simulink subsystem "FOC"  (R2023b)
settings: Solver=VariableStepAuto  StartTime=0.0  StopTime=10.0  RelTol=1e-3
undefined symbols (not defined in the file): NPoles, tSimMoCo
libraries: slpidlib x2
settings Model: Creator=Elio  LastModifiedBy=Elio

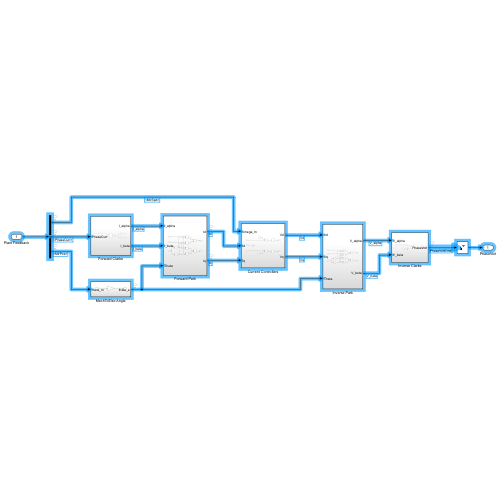
[thumbnail: Simulink's stored preview of the top-level diagram]
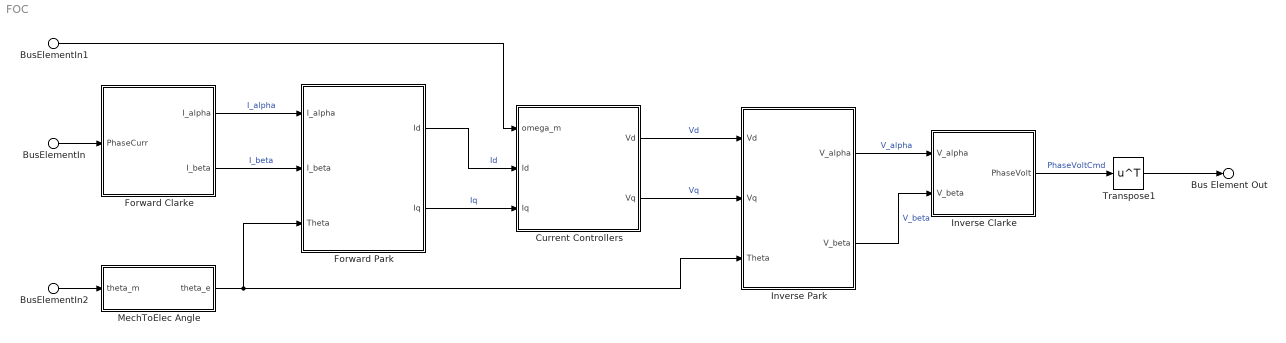
== system FOC ==
  BusElementIn1 : Inport  PortName=FOCInputs  Element=wRotorSpd
  BusElementIn : Inport  PortName=FOCInputs  Element=IPhase
  BusElementIn2 : Inport  PortName=FOCInputs  Element=aRotorMechPos
  Current Controllers : Subsystem
  Forward Clarke : Subsystem
  Forward Park : Subsystem
  Inverse Clarke : Subsystem
  Inverse Park : Subsystem
  MechToElec Angle : Subsystem
  Transpose1 : Math  Operator=transpose
  Bus Element Out : Outport  PortName=FOCCmds  Element=VPhase
  wires:
  Current Controllers/1(Vd) -> Inverse Park/1(Vd)  "Vd"
  Forward Clarke/2(I_beta) -> Forward Park/2(I_beta)  "I_beta"
  Current Controllers/2(Vq) -> Inverse Park/2(Vq)  "Vq"
  Forward Park/1(Id) -> Current Controllers/2(Id)  "Id"
  MechToElec Angle/1(theta_e) -> Forward Park/3(Theta), Inverse Park/3(Theta)
  BusElementIn/1 -> Forward Clarke/1(PhaseCurr)
  Forward Clarke/1(I_alpha) -> Forward Park/1(I_alpha)  "I_alpha"
  Inverse Park/2(V_beta) -> Inverse Clarke/2(V_beta)  "V_beta"
  Inverse Park/1(V_alpha) -> Inverse Clarke/1(V_alpha)  "V_alpha"
  Transpose1/1 -> Bus Element Out/1
  Forward Park/2(Iq) -> Current Controllers/3(Iq)  "Iq"
  Inverse Clarke/1(PhaseVolt) -> Transpose1/1  "PhaseVoltCmd"
  BusElementIn2/1 -> MechToElec Angle/1(theta_m)
  BusElementIn1/1 -> Current Controllers/1(omega_m)

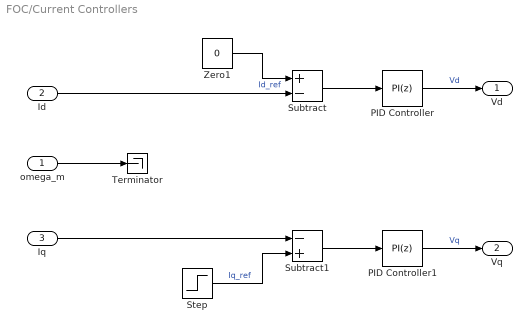
== system FOC/Current Controllers ==
  omega_m : Inport
  Id : Inport  Port=2
  Iq : Inport  Port=3
  PID Controller : slpidlib/PID Controller  Controller=PI  Form=Parallel  TimeDomain=Discrete-time  UseExternalTs=off  SampleTime=1e-5  IntegratorMethod=Forward Euler  FilterMethod=Forward Euler  ControllerParametersSource=internal  P=13.4666695236978  I=8567.48164264561  UseKiTs=off  D=0  N=100  UseFilter=on  TunerSelectOption=Transfer Function Based (PID Tuner App)  InitialConditionSource=internal  InitialConditionForIntegrator=0  InitialConditionForFilter=0  DifferentiatorICPrevScaledInput=0  ExternalReset=none  TrackingMode=off  Kt=1  LimitOutput=off  SatLimitsSource=internal  UpperSaturationLimit=inf  LowerSaturationLimit=-inf  LinearizeAsGain=on  AntiWindupMode=none  Kb=1  LimitIntegrator=off  UpperIntegratorSaturationLimit=inf  LowerIntegratorSaturationLimit=-inf  POutMin=[]  POutMax=[]  IOutMin=[]  IOutMax=[]  DOutMin=[]  DOutMax=[]  NOutMin=[]  NOutMax=[]  SumOutMin=[]  SumOutMax=[]  SaturationOutMin=[]  SaturationOutMax=[]  PParamMin=[]  PParamMax=[]  IParamMin=[]  IParamMax=[]  DParamMin=[]  DParamMax=[]  NParamMin=[]  NParamMax=[]  KbParamMin=[]  KbParamMax=[]  KtParamMin=[]  KtParamMax=[]  KbOutMin=[]  KbOutMax=[]  KtOutMin=[]  KtOutMax=[]  IntegratorOutMin=[]  IntegratorOutMax=[]  FilterOutMin=[]  FilterOutMax=[]  SumI1OutMin=[]  SumI1OutMax=[]  SumI2OutMin=[]  SumI2OutMax=[]  SumI3OutMin=[]  SumI3OutMax=[]  SumI4OutMin=[]  SumI4OutMax=[]  SumDOutMin=[]  SumDOutMax=[]  DifferentiatorOutMin=[]  DifferentiatorOutMax=[]  FilterDiffOutCoefMin=[]  FilterDiffOutCoefMax=[]  ReciprocalOutMin=[]  ReciprocalOutMax=[]  SumDenOutMin=[]  SumDenOutMax=[]  SumNumOutMin=[]  SumNumOutMax=[]  DivideOutMin=[]  DivideOutMax=[]  UdiffTsProdOutMin=[]  UdiffTsProdOutMax=[]  NTsProdOutMin=[]  NTsProdOutMax=[]  UintegralTsProdOutMin=[]  UintegralTsProdOutMax=[]  UngainTsProdOutMin=[]  UngainTsProdOutMax=[]  ClampingZeroOutDataTypeStr=Inherit: Inherit via back propagation  ClampingZeroOutMin=[]  ClampingZeroOutMax=[]  FilterDenConstantOutDataTypeStr=Inherit: Inherit via back propagation  FilterDenConstantOutMin=[]  FilterDenConstantOutMax=[]  PCopyOutDataTypeStr=Inherit: Inherit via back propagation  PCopyOutMin=[]  PCopyOutMax=[]  NCopyOutDataTypeStr=Inherit: Inherit via back propagation  NCopyOutMin=[]  NCopyOutMax=[]  IntegratorContinuousStateAttributes=''  IntegratorStateMustResolveToSignalObject=off  IntegratorRTWStateStorageClass=Auto  FilterContinuousStateAttributes=''  FilterStateMustResolveToSignalObject=off  FilterRTWStateStorageClass=Auto  ParallelPVariant=InternalParameters  IdealPVariant=Disabled  IVariant=InternalParameters  DVariant=Disabled  IntegratorVariant=Discrete  SatVariant=Disabled  AWVariant=Passthrough  PCopyVariant=Disabled  TRVariant=Disabled  FdbkBlocksVariant=Forward  IdealPFdbkVariant=Disabled  SatFdbkVariant=Disabled  DerivativeFilterVariant=Disabled  NVariant=Disabled  NCopyVariant=Disabled_SignalSpec  FilterICVariant=Disabled  IntegratorICVariant=InternalICs  ExternalResetVariant=Disabled  TRSumVariant=Passthrough  SumFdbkVariant=Disabled  SumVariant=Sum_PI  TsampFilterVariant=InternalTs  TsampNgainVariant=Passthrough  TsampIntegralVariant=Disabled_SignalSpec  ExternalSaturationOutDataTypeStr=Inherit: Same as second input
  PID Controller1 : slpidlib/PID Controller  Controller=PI  Form=Parallel  TimeDomain=Discrete-time  UseExternalTs=off  SampleTime=1e-5  IntegratorMethod=Forward Euler  FilterMethod=Forward Euler  ControllerParametersSource=internal  P=25  I=12500  UseKiTs=off  D=0  N=100  UseFilter=on  TunerSelectOption=Transfer Function Based (PID Tuner App)  InitialConditionSource=internal  InitialConditionForIntegrator=0  InitialConditionForFilter=0  DifferentiatorICPrevScaledInput=0  ExternalReset=none  TrackingMode=off  Kt=1  LimitOutput=off  SatLimitsSource=internal  UpperSaturationLimit=inf  LowerSaturationLimit=-inf  LinearizeAsGain=on  AntiWindupMode=none  Kb=1  LimitIntegrator=off  UpperIntegratorSaturationLimit=inf  LowerIntegratorSaturationLimit=-inf  POutMin=[]  POutMax=[]  IOutMin=[]  IOutMax=[]  DOutMin=[]  DOutMax=[]  NOutMin=[]  NOutMax=[]  SumOutMin=[]  SumOutMax=[]  SaturationOutMin=[]  SaturationOutMax=[]  PParamMin=[]  PParamMax=[]  IParamMin=[]  IParamMax=[]  DParamMin=[]  DParamMax=[]  NParamMin=[]  NParamMax=[]  KbParamMin=[]  KbParamMax=[]  KtParamMin=[]  KtParamMax=[]  KbOutMin=[]  KbOutMax=[]  KtOutMin=[]  KtOutMax=[]  IntegratorOutMin=[]  IntegratorOutMax=[]  FilterOutMin=[]  FilterOutMax=[]  SumI1OutMin=[]  SumI1OutMax=[]  SumI2OutMin=[]  SumI2OutMax=[]  SumI3OutMin=[]  SumI3OutMax=[]  SumI4OutMin=[]  SumI4OutMax=[]  SumDOutMin=[]  SumDOutMax=[]  DifferentiatorOutMin=[]  DifferentiatorOutMax=[]  FilterDiffOutCoefMin=[]  FilterDiffOutCoefMax=[]  ReciprocalOutMin=[]  ReciprocalOutMax=[]  SumDenOutMin=[]  SumDenOutMax=[]  SumNumOutMin=[]  SumNumOutMax=[]  DivideOutMin=[]  DivideOutMax=[]  UdiffTsProdOutMin=[]  UdiffTsProdOutMax=[]  NTsProdOutMin=[]  NTsProdOutMax=[]  UintegralTsProdOutMin=[]  UintegralTsProdOutMax=[]  UngainTsProdOutMin=[]  UngainTsProdOutMax=[]  ClampingZeroOutDataTypeStr=Inherit: Inherit via back propagation  ClampingZeroOutMin=[]  ClampingZeroOutMax=[]  FilterDenConstantOutDataTypeStr=Inherit: Inherit via back propagation  FilterDenConstantOutMin=[]  FilterDenConstantOutMax=[]  PCopyOutDataTypeStr=Inherit: Inherit via back propagation  PCopyOutMin=[]  PCopyOutMax=[]  NCopyOutDataTypeStr=Inherit: Inherit via back propagation  NCopyOutMin=[]  NCopyOutMax=[]  IntegratorContinuousStateAttributes=''  IntegratorStateMustResolveToSignalObject=off  IntegratorRTWStateStorageClass=Auto  FilterContinuousStateAttributes=''  FilterStateMustResolveToSignalObject=off  FilterRTWStateStorageClass=Auto  ParallelPVariant=InternalParameters  IdealPVariant=Disabled  IVariant=InternalParameters  DVariant=Disabled  IntegratorVariant=Discrete  SatVariant=Disabled  AWVariant=Passthrough  PCopyVariant=Disabled  TRVariant=Disabled  FdbkBlocksVariant=Forward  IdealPFdbkVariant=Disabled  SatFdbkVariant=Disabled  DerivativeFilterVariant=Disabled  NVariant=Disabled  NCopyVariant=Disabled_SignalSpec  FilterICVariant=Disabled  IntegratorICVariant=InternalICs  ExternalResetVariant=Disabled  TRSumVariant=Passthrough  SumFdbkVariant=Disabled  SumVariant=Sum_PI  TsampFilterVariant=InternalTs  TsampNgainVariant=Passthrough  TsampIntegralVariant=Disabled_SignalSpec  ExternalSaturationOutDataTypeStr=Inherit: Same as second input
  Step : Step  After=10  SampleTime=tSimMoCo
  Subtract : Sum  Inputs=+-
  Subtract1 : Sum  Inputs=-+
  Terminator : Terminator
  Zero1 : Constant  Value=0  OutDataTypeStr=Inherit: Inherit via back propagation  SampleTime=tSimMoCo
  Vd : Outport
  Vq : Outport  Port=2
  wires:
  Subtract1/1 -> PID Controller1/1
  Step/1 -> Subtract1/2  "Iq_ref"
  Zero1/1 -> Subtract/1  "Id_ref"
  Subtract/1 -> PID Controller/1
  Id/1 -> Subtract/2
  Iq/1 -> Subtract1/1
  PID Controller/1 -> Vd/1  "Vd"
  PID Controller1/1 -> Vq/1  "Vq"
  omega_m/1 -> Terminator/1

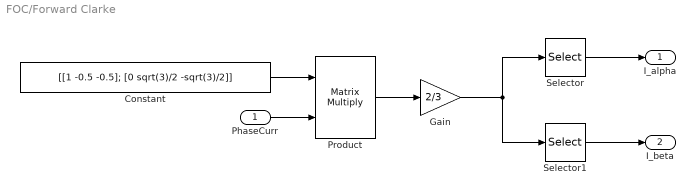
== system FOC/Forward Clarke ==
  PhaseCurr : Inport
  Constant : Constant  Value=[[1 -0.5 -0.5]; [0 sqrt(3)/2 -sqrt(3)/2]]  SampleTime=tSimMoCo
  Gain : Gain  Gain=2/3
  Product : Product  Multiplication=Matrix(*)
  Selector : Selector  InputPortWidth=2  IndexOptions=Index vector (dialog)  Indices=1  OutputSizes=1
  Selector1 : Selector  InputPortWidth=2  IndexOptions=Index vector (dialog)  Indices=2  OutputSizes=1
  I_alpha : Outport
  I_beta : Outport  Port=2
  wires:
  Constant/1 -> Product/1
  Product/1 -> Gain/1
  Gain/1 -> Selector1/1, Selector/1
  Selector/1 -> I_alpha/1
  Selector1/1 -> I_beta/1
  PhaseCurr/1 -> Product/2

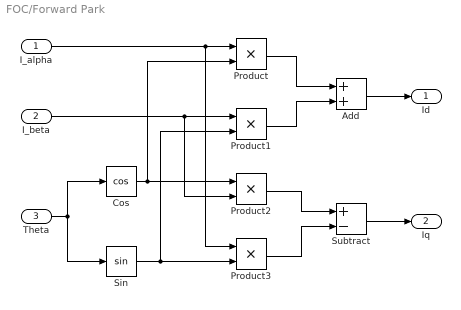
== system FOC/Forward Park ==
  I_alpha : Inport
  I_beta : Inport  Port=2
  Theta : Inport  Port=3
  Add : Sum
  Cos : Trigonometry  Operator=cos
  Product{,1..3} (4 alike) : Product
  Sin : Trigonometry
  Subtract : Sum  Inputs=+-
  Id : Outport
  Iq : Outport  Port=2
  wires:
  Theta/1 -> Sin/1, Cos/1
  I_alpha/1 -> Product/1, Product3/1
  Cos/1 -> Product2/1, Product/2
  I_beta/1 -> Product1/1, Product2/2
  Sin/1 -> Product3/2, Product1/2
  Product/1 -> Add/1
  Product1/1 -> Add/2
  Add/1 -> Id/1
  Product2/1 -> Subtract/1
  Product3/1 -> Subtract/2
  Subtract/1 -> Iq/1

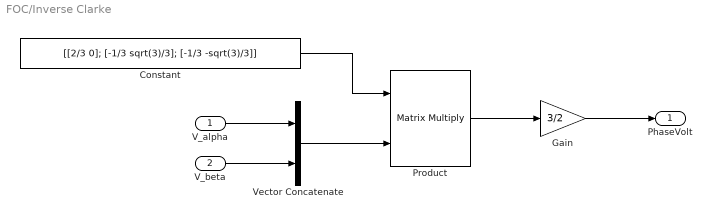
== system FOC/Inverse Clarke ==
  V_alpha : Inport
  V_beta : Inport  Port=2
  Constant : Constant  Value=[[2/3 0]; [-1/3 sqrt(3)/3]; [-1/3 -sqrt(3)/3]]  SampleTime=tSimMoCo
  Gain : Gain  Gain=3/2
  Product : Product  Multiplication=Matrix(*)
  Vector Concatenate : Concatenate
  PhaseVolt : Outport
  wires:
  V_alpha/1 -> Vector Concatenate/1
  V_beta/1 -> Vector Concatenate/2
  Vector Concatenate/1 -> Product/2
  Constant/1 -> Product/1
  Product/1 -> Gain/1
  Gain/1 -> PhaseVolt/1

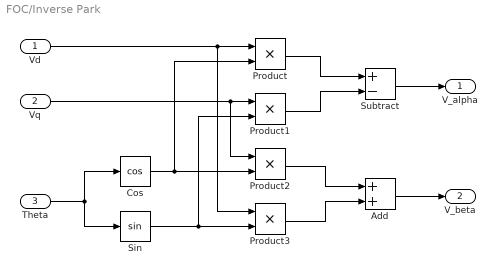
== system FOC/Inverse Park ==
  Vd : Inport
  Vq : Inport  Port=2
  Theta : Inport  Port=3
  Add : Sum
  Cos : Trigonometry  Operator=cos
  Product{,1..3} (4 alike) : Product
  Sin : Trigonometry
  Subtract : Sum  Inputs=+-
  V_alpha : Outport
  V_beta : Outport  Port=2
  wires:
  Theta/1 -> Cos/1, Sin/1
  Vd/1 -> Product3/1, Product/1
  Cos/1 -> Product/2, Product2/2
  Vq/1 -> Product2/1, Product1/1
  Sin/1 -> Product1/2, Product3/2
  Product/1 -> Subtract/1
  Product1/1 -> Subtract/2
  Subtract/1 -> V_alpha/1
  Product2/1 -> Add/1
  Product3/1 -> Add/2
  Add/1 -> V_beta/1

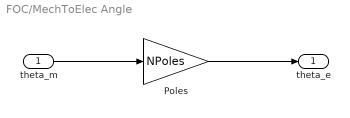
== system FOC/MechToElec Angle ==
  theta_m : Inport
  Poles : Gain  Gain=NPoles
  theta_e : Outport
  wires:
  theta_m/1 -> Poles/1
  Poles/1 -> theta_e/1
